simulink model "task_03"  (R2024b)
settings: Solver=VariableStepAuto  StartTime=0.0  StopTime=10.0  RelTol=1e-3
settings Model: Creator=jx2004  LastModifiedBy=jx2004

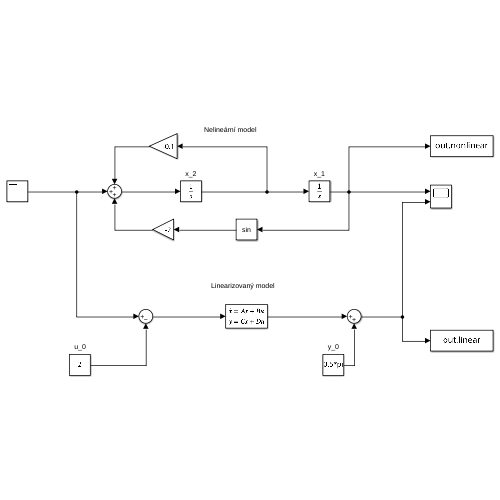
[thumbnail: Simulink's stored preview of the top-level diagram]
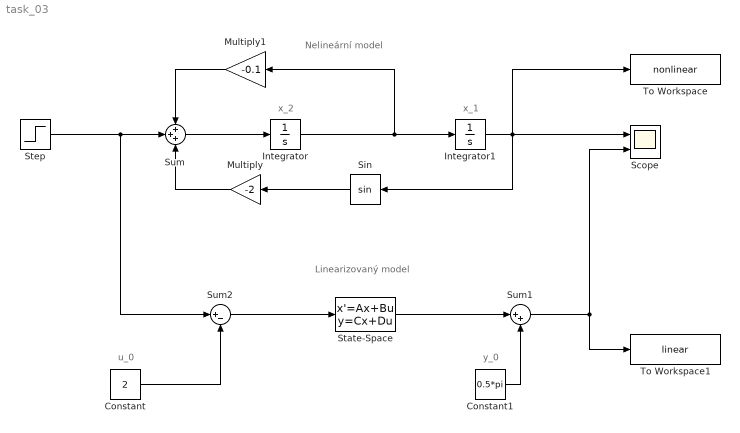
== system task_03 ==
  note: Nelineární model
  note: Linearizovaný model
  note: y_0
  note: u_0
  note: x_1
  note: x_2
  Constant : Constant  Value=2
  Constant1 : Constant  Value=0.5*pi
  Integrator : Integrator
  Integrator1 : Integrator  InitialCondition=pi/2
  Multiply : Gain  Gain=-2
  Multiply1 : Gain  Gain=-0.1
  Scope : Scope  NumInputPorts=2
  Sin : Trigonometry
  State-Space : StateSpace  A=[0 1; 0 -0.1]  B=[0; 1]  C=[1 0]  D=0  InitialCondition=0
  Step : Step  Before=2  SampleTime=0
  Sum : Sum  Inputs=+++
  Sum1 : Sum  Inputs=|++
  Sum2 : Sum  Inputs=|+-
  To Workspace : ToWorkspace  VariableName=nonlinear  SaveFormat=Timeseries  SampleTime=-1
  To Workspace1 : ToWorkspace  VariableName=linear  SaveFormat=Timeseries  SampleTime=-1
  wires:
  Sum2/1 -> State-Space/1
  Constant/1 -> Sum2/2
  Sin/1 -> Multiply/1
  Multiply/1 -> Sum/3
  Multiply1/1 -> Sum/1
  Sum/1 -> Integrator/1
  Integrator/1 -> Integrator1/1, Multiply1/1
  Integrator1/1 -> To Workspace/1, Scope/1, Sin/1
  State-Space/1 -> Sum1/1
  Constant1/1 -> Sum1/2
  Sum1/1 -> Scope/2, To Workspace1/1
  Step/1 -> Sum2/1, Sum/2
